simulink subsystem "matlabMotorModelTest"  (R2024b)
settings: Solver=VariableStepAuto  StartTime=0.0  StopTime=10.0  RelTol=1e-3
settings Model: Creator=aborawake  LastModifiedBy=aborawake

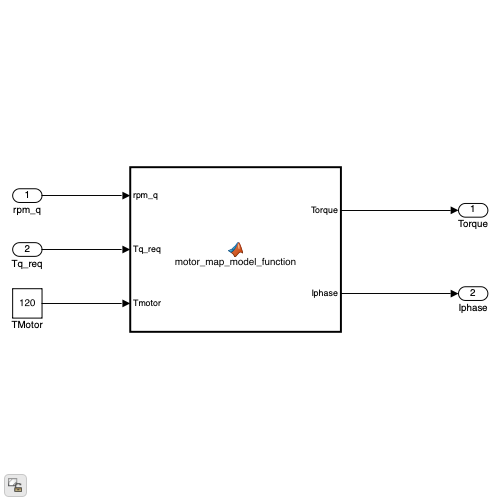
[thumbnail: Simulink's stored preview of the top-level diagram]
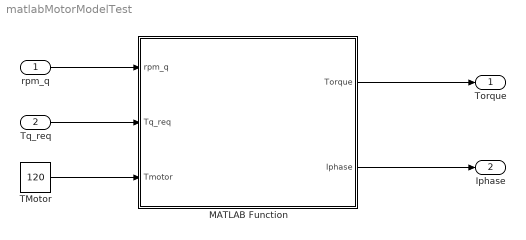
== system matlabMotorModelTest ==
  rpm_q : Inport
  Tq_req : Inport  Port=2
  MATLAB Function : MATLAB Function  TreatAsAtomicUnit=on
  TMotor : Constant  Value=120
  Torque : Outport
  Iphase : Outport  Port=2
  wires:
  MATLAB Function/1(Torque) -> Torque/1
  MATLAB Function/2(Iphase) -> Iphase/1
  rpm_q/1 -> MATLAB Function/1(rpm_q)
  Tq_req/1 -> MATLAB Function/2(Tq_req)
  TMotor/1 -> MATLAB Function/3(Tmotor)

== matlab function matlabMotorModelTest/MATLAB Function ==
  data: rpm_q input; Tq_req input; Tmotor input; Torque output; Iphase output
function [Torque, Iphase] =  motor_map_model_function(rpm_q, Tq_req, Tmotor)
% Inputs:
%   rpm_q   - mechanical speed [rpm]
%   Tq_req  - torque request [Nm]
%   Tmotor  - motor temperature [°C]
%   maps80  - struct of griddedInterpolants (80 °C)
%   maps120 - struct of griddedInterpolants (120 °C)
%   limits  - struct with fields:
%                I_max, V_dc, V_margin
% Outputs:
%   out struct with fields: Iq, Id, Iphase, Vd, Vq, Torque, Ploss
    
    % Datasheet constants
    p       = 5;           % pole pairs
    R_s     = 0.135;       % stator resistance [ohm]
    Ld      = 0.24e-3;     % [H]
    Lq      = 0.12e-3;     % [H]
    kt      = 0.26;        % Nm/Arms
    J       = 2.74e-4;     % [kg*m^2]


    limits.I_max   = 105;         % Arms
    limits.V_dc    = 350;         % V (nominal DC bus)
    limits.V_margin= 30;          % V reserve margin

    % Load MAT files
    data80  = load('A2370DD_T80C.mat');
    data100 = load('A2370DD_T100C.mat');
    data120 = load('A2370DD_T120C.mat');
    
    % Axes setup (hopefully this is right)
    rpm_vec = data100.Speed(:,1);          
    T_vec   = data100.Shaft_Torque(1,:);   
    
    % Build gridded interpolnts
    fields = {'Shaft_Torque','Id_RMS','Iq_RMS','Stator_Current_Phase_RMS',...
              'Vd_RMS','Vq_RMS','Total_Loss','Stator_Copper_Loss',...
              'Iron_Loss','Magnet_Loss','Mechanical_Loss'};
    
    maps80 = struct(); maps100 = struct(); maps120 = struct();
    
    for i = 1:length(fields)
        f = fields{i};
        maps80.(f)  = griddedInterpolant({rpm_vec, T_vec}, data80.(f),  'linear','nearest');
        maps100.(f) = griddedInterpolant({rpm_vec, T_vec}, data100.(f), 'linear','nearest');
        maps120.(f) = griddedInterpolant({rpm_vec, T_vec}, data120.(f), 'linear','nearest');
    end




    
    alpha = max(0,min(1,(Tmotor-80)/(120-80)));
    % Interpolated values
    Iq_val = (1-alpha)*maps80.Iq_RMS(rpm_q,Tq_req)   + alpha*maps120.Iq_RMS(rpm_q,Tq_req);
    Id_val = (1-alpha)*maps80.Id_RMS(rpm_q,Tq_req)   + alpha*maps120.Id_RMS(rpm_q,Tq_req);
    Iphase = (1-alpha)*maps80.Stator_Current_Phase_RMS(rpm_q,Tq_req) ...
                    + alpha*maps120.Stator_Current_Phase_RMS(rpm_q,Tq_req);
    Vd_val = (1-alpha)*maps80.Vd_RMS(rpm_q,Tq_req)   + alpha*maps120.Vd_RMS(rpm_q,Tq_req);
    Vq_val = (1-alpha)*maps80.Vq_RMS(rpm_q,Tq_req)   + alpha*maps120.Vq_RMS(rpm_q,Tq_req);
    Torque = (1-alpha)*maps80.Shaft_Torque(rpm_q,Tq_req) + alpha*maps120.Shaft_Torque(rpm_q,Tq_req);
    Ploss  = (1-alpha)*maps80.Total_Loss(rpm_q,Tq_req)   + alpha*maps120.Total_Loss(rpm_q,Tq_req);

    % Current limit
    if Iphase > limits.I_max
        scale   = limits.I_max / Iphase;
        Iq_val  = Iq_val*scale; 
        Id_val  = Id_val*scale;
        Torque  = Torque*scale;
        Iphase  = limits.I_max;
    end

    % Voltage limit
    V_lim = (limits.V_dc - limits.V_margin)/sqrt(3);
    V_req = sqrt(Vd_val^2 + Vq_val^2);
    if V_req > V_lim
        Torque = Torque * (V_lim/V_req);
    end


    Torque = Torque*14.33;

    % Pack output
    out.Iq = Iq_val;
    out.Id = Id_val;
    out.Iphase = Iphase;
    out.Vd = Vd_val;
    out.Vq = Vq_val;
    out.Torque = Torque;
    out.Ploss = Ploss;
    out.Vreq = V_req;
end
